simulink model "mod3_CRFF_DTExample"  (Simulink 8.9)
settings: Solver=VariableStepDiscrete  StartTime=0.0  StopTime=simu.trantime  RelTol=1e-3  EnableMultiTasking=on
values from neighbouring files (symbols this model uses):
  Fs = fb*2*OSR    (= 6144000)    [CRFF_DTExample.m]
undefined symbols (not defined in the file or in its folder): a, b, c, g, mod
libraries: dspsrcs4 x1
settings Model: Creator=amyles  LastModifiedBy=Arnaldi Isacco
settings DataIOCC: MaxDataPoints=50000
settings OptimizationCC: DefaultParameterBehavior=Inlined  ExpressionDepthLimit=2147483647
settings DebuggingCC: UnderspecifiedInitializationDetection=Simplified  MergeDetectMultiDrivingBlocksExec=error  SolverPrmCheckMsg=warning  InvalidFcnCallConnMsg=warning  StrictBusMsg=ErrorOnBusTreatedAsVector
settings ModelReferenceCC: ModelReferenceNumInstancesAllowed=Single

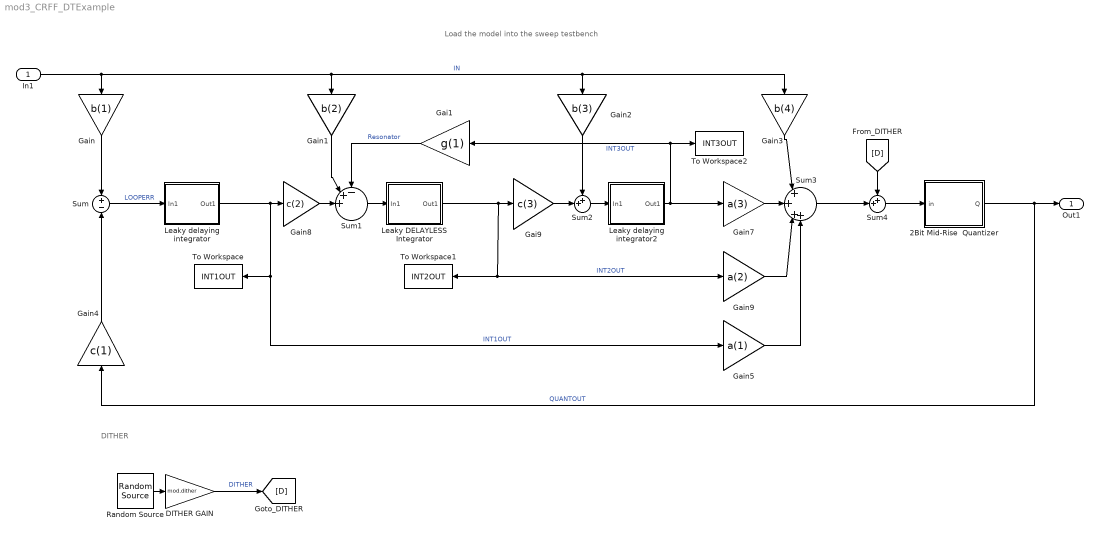
== system mod3_CRFF_DTExample ==
  note: DITHER
  note: Load the model into the sweep testbench
  In1 : Inport
  2Bit Mid-Rise  Quantizer : Subsystem
  DITHER GAIN : Gain  Gain=mod.dither
  Gai1 : Gain  Gain=g(1)
  Gai9 : Gain  Gain=c(3)
  Gain : Gain  Gain=b(1)  SampleTime=1/Fs
  Gain1 : Gain  Gain=b(2)  SampleTime=1/Fs
  Gain2 : Gain  Gain=b(3)  SampleTime=1/Fs
  Gain3 : Gain  Gain=b(4)  SampleTime=1/Fs
  Gain4 : Gain  Gain=c(1)  SampleTime=1/Fs
  Gain5 : Gain  Gain=a(1)
  Gain7 : Gain  Gain=a(3)
  Gain8 : Gain  Gain=c(2)
  Gain9 : Gain  Gain=a(2)
  Leaky DELAYLESS Integrator : Subsystem
  Leaky delaying integrator : Subsystem
  Leaky delaying integrator2 : Subsystem
  Random Source : dspsrcs4/Random Source  SrcType=Uniform  NormMethod=Ziggurat  CltLength=12  MinVal=-1  MaxVal=1  MeanVal=0  VarVal=1  RepMode=Not repeatable  rawSeed=1  IsInherit=off  SampMode=Discrete  SampTime=1/Fs  SampFrame=1  DataType=Double  OutComplex=Real  OutputFrames=on
  Sum : Sum  Inputs=+-  SampleTime=1/Fs
  Sum1 : Sum  Inputs=-++||
  Sum2 : Sum  Inputs=++|
  Sum3 : Sum  Inputs=|+|+|++
  Sum4 : Sum  Inputs=++|
  To Workspace : ToWorkspace  VariableName=INT1OUT  SampleTime=-1
  To Workspace1 : ToWorkspace  VariableName=INT2OUT  SampleTime=-1
  To Workspace2 : ToWorkspace  VariableName=INT3OUT  SampleTime=-1
  Out1 : Outport
  wires:
  In1/1 -> Gain3/1, Gain2/1, Gain1/1, Gain/1  "IN"
  Gain8/1 -> Sum1/3
  Leaky DELAYLESS Integrator/1(Out1) -> Gai9/1, Gain9/1, To Workspace1/1  "INT2OUT"
  Gai9/1 -> Sum2/2
  Leaky delaying integrator2/1(Out1) -> Gain7/1, To Workspace2/1, Gai1/1  "INT3OUT"
  Gain4/1 -> Sum/2
  Gain/1 -> Sum/1
  Gain1/1 -> Sum1/2
  Gai1/1 -> Sum1/1  "Resonator"
  Gain2/1 -> Sum2/1
  2Bit Mid-Rise  Quantizer/1(Q) -> Out1/1, Gain4/1  "QUANTOUT"
  Sum/1 -> Leaky delaying integrator/1(In1)  "LOOPERR"
  Sum2/1 -> Leaky delaying integrator2/1(In1)
  Sum1/1 -> Leaky DELAYLESS Integrator/1(In1)
  Gain3/1 -> Sum3/1
  Gain7/1 -> Sum3/2
  Gain9/1 -> Sum3/3
  Gain5/1 -> Sum3/4
  Random Source/1 -> DITHER GAIN/1
  DITHER GAIN/1 -> [D]  "DITHER"
  Leaky delaying integrator/1(Out1) -> Gain8/1, Gain5/1, To Workspace/1  "INT1OUT"
  [D] -> Sum4/1
  Sum3/1 -> Sum4/2
  Sum4/1 -> 2Bit Mid-Rise  Quantizer/1(in)

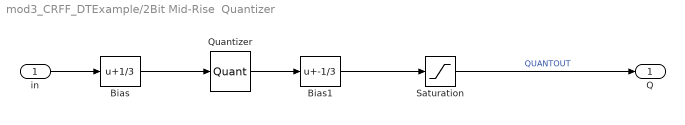
== system mod3_CRFF_DTExample/2Bit Mid-Rise  Quantizer ==
  in : Inport
  Bias : Bias  Bias=1/3
      settings: AttributesFormatString=Need offset to give\nMID-RISE quantiser
  Bias1 : Bias  Bias=-1/3
  Quantizer : Quantizer  QuantizationInterval=2/3  LinearizeAsGain=off  SampleTime=1/Fs
  Saturation : Saturate  UpperLimit=mod.qsatout1  LowerLimit=-(mod.qsatout1)
  Q : Outport
  wires:
  Bias/1 -> Quantizer/1
  Saturation/1 -> Q/1  "QUANTOUT"
  Quantizer/1 -> Bias1/1
  Bias1/1 -> Saturation/1
  in/1 -> Bias/1

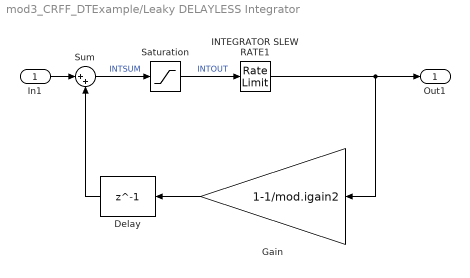
== system mod3_CRFF_DTExample/Leaky DELAYLESS Integrator ==
  In1 : Inport
  Delay : Delay  DelayLength=1  InitialCondition=0  InputProcessing=Inherited
  Gain : Gain  Gain=1-1/mod.igain2
      settings: AttributesFormatString=Integrator leakage
  INTEGRATOR SLEW RATE1 : RateLimiter  RisingSlewLimit=mod.isr2  FallingSlewLimit=-(mod.isr2)  SampleTimeMode=inherited
  Saturation : Saturate  UpperLimit=mod.isat2  LowerLimit=-(mod.isat2)
  Sum : Sum  Inputs=|++
      settings: AttributesFormatString=Integrator summer
  Out1 : Outport
  wires:
  In1/1 -> Sum/1
  Gain/1 -> Delay/1
  Sum/1 -> Saturation/1  "INTSUM"
  Delay/1 -> Sum/2
  Saturation/1 -> INTEGRATOR SLEW RATE1/1  "INTOUT"
  INTEGRATOR SLEW RATE1/1 -> Gain/1, Out1/1

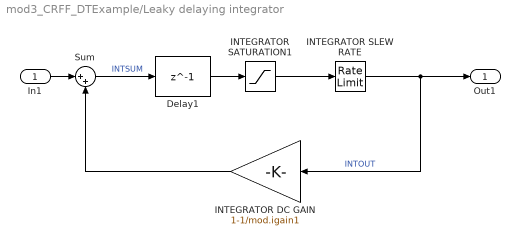
== system mod3_CRFF_DTExample/Leaky delaying integrator ==
  In1 : Inport
  Delay1 : Delay  DelayLength=1  InitialCondition=0  InputProcessing=Inherited
  INTEGRATOR SATURATION1 : Saturate  UpperLimit=mod.isat1  LowerLimit=-(mod.isat1)
  INTEGRATOR SLEW RATE : RateLimiter  RisingSlewLimit=mod.isr1  FallingSlewLimit=-(mod.isr1)  SampleTimeMode=inherited
  INTEGRATOR DC GAIN : Gain  Gain=1-1/mod.igain1
      settings: AttributesFormatString=Integrator leakage\n(model finite integrator dc/LF\ngain in analog modulators)
  Sum : Sum  Inputs=|++  SampleTime=1/Fs
      settings: AttributesFormatString=Integrator summer
  Out1 : Outport
  wires:
  Sum/1 -> Delay1/1  "INTSUM"
  INTEGRATOR DC GAIN/1 -> Sum/2
  INTEGRATOR SATURATION1/1 -> INTEGRATOR SLEW RATE/1
  In1/1 -> Sum/1
  Delay1/1 -> INTEGRATOR SATURATION1/1
  INTEGRATOR SLEW RATE/1 -> Out1/1, INTEGRATOR DC GAIN/1  "INTOUT"

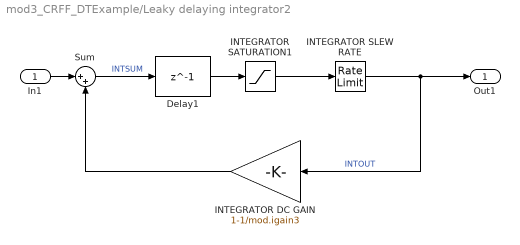
== system mod3_CRFF_DTExample/Leaky delaying integrator2 ==
  In1 : Inport
  Delay1 : Delay  DelayLength=1  InitialCondition=0  InputProcessing=Inherited
  INTEGRATOR SATURATION1 : Saturate  UpperLimit=mod.isat3  LowerLimit=-(mod.isat3)
  INTEGRATOR SLEW RATE : RateLimiter  RisingSlewLimit=mod.isr3  FallingSlewLimit=-(mod.isr3)  SampleTimeMode=inherited
  INTEGRATOR DC GAIN : Gain  Gain=1-1/mod.igain3
      settings: AttributesFormatString=Integrator leakage\n(model finite integrator dc/LF\ngain in analog modulators)
  Sum : Sum  Inputs=|++
      settings: AttributesFormatString=Integrator summer
  Out1 : Outport
  wires:
  Sum/1 -> Delay1/1  "INTSUM"
  INTEGRATOR DC GAIN/1 -> Sum/2
  INTEGRATOR SATURATION1/1 -> INTEGRATOR SLEW RATE/1
  In1/1 -> Sum/1
  Delay1/1 -> INTEGRATOR SATURATION1/1
  INTEGRATOR SLEW RATE/1 -> Out1/1, INTEGRATOR DC GAIN/1  "INTOUT"
